simulink model "RCAM_Geodetic"  (R2024b)
settings: Solver=VariableStepAuto  StartTime=0.0  StopTime=10.0  RelTol=1e-3
values from neighbouring files (symbols this model uses):
  u1max = 25*pi/180    (= 0.436332312999)    [RCAM_model.m]
  u1min = -25*pi/180    (= -0.436332312999)    [RCAM_model.m]
  u2max = 10*pi/180    (= 0.174532925199)    [RCAM_model.m]
  u2min = -25*pi/180    (= -0.436332312999)    [RCAM_model.m]
  u3max = 30*pi/180    (= 0.523598775598)    [RCAM_model.m]
  u3min = - 30*pi/180    (= -0.523598775598)    [RCAM_model.m]
  u4max = 10*pi/180    (= 0.174532925199)    [RCAM_model.m]
  u5max = 10*pi/180    (= 0.174532925199)    [RCAM_model.m]
  u5min = 0.5*pi/180    (= 0.00872664625997)    [RCAM_model.m]
  x0 = [85 ... (first row only)    [sim_initialise.m]
undefined symbols (not defined in the file or in its folder): RCAM_model_new, u14min
libraries: AE512Blockset x2
settings Model: Creator=satvik_sh  LastModifiedBy=satvik_sh

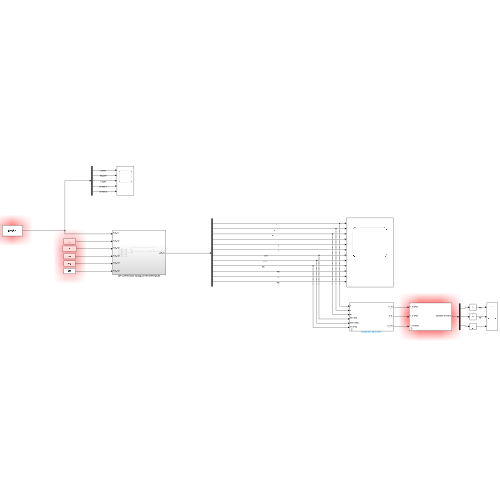
[thumbnail: Simulink's stored preview of the top-level diagram]
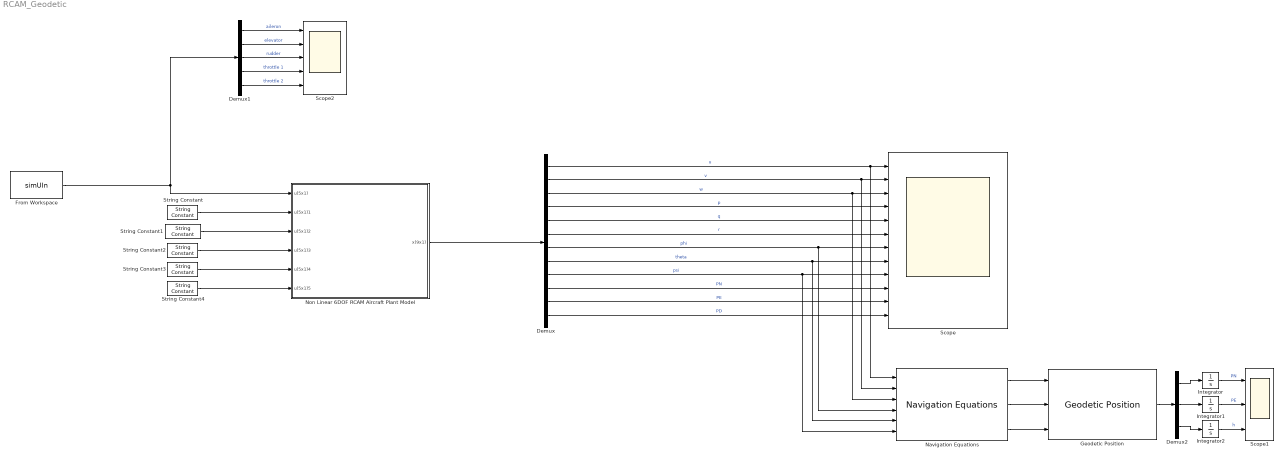
== system RCAM_Geodetic ==
  Demux : Demux  Outputs=12
  Demux1 : Demux  Outputs=5
  Demux2 : Demux  Outputs=3
  From Workspace : FromWorkspace  VariableName=simUIn
  Geodetic Position : AE512Blockset/Geodetic Position  Xgeodetic0=Xgeodetic0
  Integrator : Integrator
  Integrator1 : Integrator
  Integrator2 : Integrator
  Navigation Equations : AE512Blockset/Navigation Equations  Description=|
      | Version History  
      |                  
      | 05/24/05: Created
  Non Linear 6DOF RCAM Aircraft Plant Model : Subsystem
  Scope : Scope  NumInputPorts=12
  Scope1 : Scope  NumInputPorts=3
  Scope2 : Scope  NumInputPorts=5
  String Constant : StringConstant  String=g
  String Constant1 : StringConstant  String=rho
  String Constant2 : StringConstant  String=Xcg
  String Constant3 : StringConstant  String=Ycg
  String Constant4 : StringConstant  String=Zcg
  wires:
  Integrator1/1 -> Scope1/2  "PE"
  Demux/5 -> Scope/5  "q"
  Demux/4 -> Scope/4  "p"
  Demux/12 -> Scope/12  "PD"
  String Constant/1 -> Non Linear 6DOF RCAM Aircraft Plant Model/2(u(5x1)1)
  Demux1/4 -> Scope2/4  "throttle 1"
  String Constant1/1 -> Non Linear 6DOF RCAM Aircraft Plant Model/3(u(5x1)2)
  Integrator2/1 -> Scope1/3  "h"
  String Constant3/1 -> Non Linear 6DOF RCAM Aircraft Plant Model/5(u(5x1)4)
  Demux1/2 -> Scope2/2  "elevator"
  Demux/3 -> Navigation Equations/3, Scope/3  "w"
  Demux/10 -> Scope/10  "PN"
  String Constant2/1 -> Non Linear 6DOF RCAM Aircraft Plant Model/4(u(5x1)3)
  Demux/7 -> Navigation Equations/4, Scope/7  "phi"
  Demux1/5 -> Scope2/5  "throttle 2"
  Demux/6 -> Scope/6  "r"
  Demux/9 -> Navigation Equations/6, Scope/9  "psi"
  String Constant4/1 -> Non Linear 6DOF RCAM Aircraft Plant Model/6(u(5x1)5)
  From Workspace/1 -> Demux1/1, Non Linear 6DOF RCAM Aircraft Plant Model/1(u(5x1))
  Integrator/1 -> Scope1/1  "PN"
  Demux1/3 -> Scope2/3  "rudder"
  Demux/11 -> Scope/11  "PE"
  Demux/2 -> Navigation Equations/2, Scope/2  "v"
  Non Linear 6DOF RCAM Aircraft Plant Model/1(x(9x1)) -> Demux/1
  Demux1/1 -> Scope2/1  "aileron"
  Demux/8 -> Navigation Equations/5, Scope/8  "theta"
  Demux/1 -> Navigation Equations/1, Scope/1  "u"
  Demux2/1 -> Integrator/1
  Demux2/2 -> Integrator1/1
  Demux2/3 -> Integrator2/1
  Geodetic Position/1 -> Demux2/1
  Navigation Equations/1 -> Geodetic Position/1
  Navigation Equations/2 -> Geodetic Position/2
  Navigation Equations/3 -> Geodetic Position/3

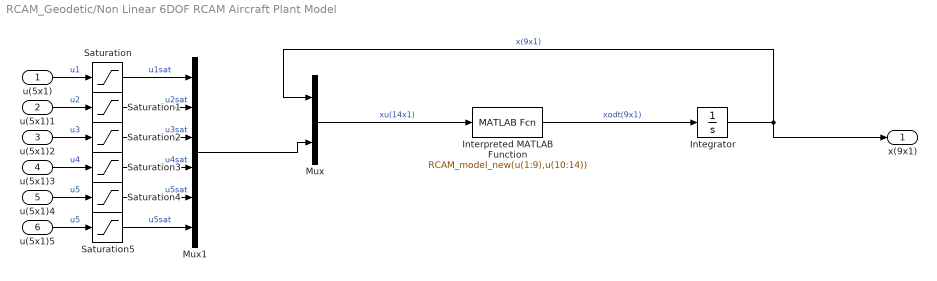
== system RCAM_Geodetic/Non Linear 6DOF RCAM Aircraft Plant Model ==
  u(5x1) : Inport
  u(5x1)1 : Inport  Port=2
  u(5x1)2 : Inport  Port=3
  u(5x1)3 : Inport  Port=4
  u(5x1)4 : Inport  Port=5
  u(5x1)5 : Inport  Port=6
  Integrator : Integrator  InitialCondition=x0
  Interpreted MATLAB Function : MATLABFcn  MATLABFcn=RCAM_model_new(u(1:9),u(10:14))
  Mux : Mux  Inputs=2
  Mux1 : Mux  Inputs=6
  Saturation : Saturate  UpperLimit=u1max  LowerLimit=u1min
  Saturation1 : Saturate  UpperLimit=u2max  LowerLimit=u2min
  Saturation2 : Saturate  UpperLimit=u3max  LowerLimit=u3min
  Saturation3 : Saturate  UpperLimit=u4max  LowerLimit=u14min
  Saturation4 : Saturate  UpperLimit=u5max  LowerLimit=u5min
  Saturation5 : Saturate  UpperLimit=u5max  LowerLimit=u5min
  x(9x1) : Outport
  wires:
  Interpreted MATLAB Function/1 -> Integrator/1  "xodt(9x1)"
  Mux/1 -> Interpreted MATLAB Function/1  "xu(14x1)"
  Integrator/1 -> x(9x1)/1, Mux/1  "x(9x1)"
  u(5x1)/1 -> Saturation/1  "u1"
  u(5x1)1/1 -> Saturation1/1  "u2"
  u(5x1)2/1 -> Saturation2/1  "u3"
  u(5x1)3/1 -> Saturation3/1  "u4"
  u(5x1)4/1 -> Saturation4/1  "u5"
  Saturation/1 -> Mux1/1  "u1sat"
  Saturation1/1 -> Mux1/2  "u2sat"
  Saturation2/1 -> Mux1/3  "u3sat"
  Saturation3/1 -> Mux1/4  "u4sat"
  Saturation4/1 -> Mux1/5  "u5sat"
  Mux1/1 -> Mux/2
  u(5x1)5/1 -> Saturation5/1  "u5"
  Saturation5/1 -> Mux1/6  "u5sat"
